simulink model "eVTOL_System"  (R2024b)
settings: Solver=FixedStepAuto  StartTime=0.0  StopTime=inf  RelTol=1e-3
undefined symbols (not defined in the file): airspeed, Battery, BCE12, BCE_Set_init, BMS_Controller_State, C, Cell10_P, Cell11_P, Cell12_P, Cell13_P, Cell14_P, Cell15_P, Cell16_P, Cell17_P, Cell18_P, Cell19_P, Cell1_N, Cell1_P, Cell20_P, Cell21_P, Cell22_P, Cell23_P, Cell24_P, Cell2_P, Cell3_P, Cell4_P, Cell5_P, Cell6_P, Cell7_P, Cell8_P, Cell9_P, Charging_State, CityMission, control, controlParams, ControlSampleTime, CriticalTiltAngle, currentFactor, CV_Gain, ddx, ddy, ddz, Device_01, Device_02, DiscIntNeverNeededParam, dx, dy, dz, Earth, env, F, F28379D_ADC_MaxCount, F28379D_ADC_Vmax, FixedWingMission, flightState, Foc_Ki_IxTcpu, Foc_Ki_S, Foc_Kp_I, Foc_Kp_S, fractalcoef ... (+68)
libraries: fl_lib x1115, nesl_utility x617, slrealtimeethercatlib x217, simulink x130, canmsglib x101, speedgoatlib_IO611_obsolete x91, slpidlib x49, mcbcontrolslib x44, slrealtimeutilitieslib x35, speedgoatlib_hdlCoder_IO3xx x31, dspstat3 x24, mcbpositiondecoderlib x12
(part 29 of 31)

== system eVTOL_System/Motor Drive/Controller/Controller_MIL/F28379D Firmware/Controller Algorithm/FOC/Current Control/Control_System/Closed Loop Control/Subsystem ==
  Iab_meas_PU : Inport
  Pos_PU : Inport  Port=2
  Idq_ref_PU : Inport  Port=3
  EnablePWM : Inport  Port=4
  Kp_i : Inport  Port=5
  Ki_ixTcpu : Inport  Port=6
  Clarke Transform : mcbcontrolslib/Clarke Transform  VariantControl=Variant2  PhaseInput=Two inputs  EnPowerInv=off
  Current_Controllers : Subsystem
  Demux : Demux  Outputs=2
  Inverse Park Transform : mcbcontrolslib/Inverse Park Transform  PhaseInput=Two inputs  AxisAlignment=D-axis  ThetaInput=Sine and Cosine electrical position  AngleInput=Per-unit  N_points=1024
  Mux : Mux
  Mux1 : Mux  Inputs=3
  Park Transform : mcbcontrolslib/Park Transform  PhaseInput=Two inputs  AxisAlignment=D-axis  ThetaInput=Sine and Cosine electrical position  AngleInput=Per-unit  N_points=1024
  Sine-Cosine Lookup : mcbcontrolslib/SinCos Embedded Optimized  LabelModeActiveChoice=MCB_Sin  OptforProc=off  ApproximationMethod=None  UserApproxMethod=Lookup  ApproxStatus=None  InterpMethod=Linear point-slope  NumberOfDataPoints=16  NumberOfIterations=11  RemoveProtectionAgainstOutOfRangeInput=off  TableDataTypeStr=Inherit: Inherit via input  AngleInput=Per-unit  ThetaDataType=single  N_points=1024  DatatypeInput=Inherit from input  Datatype=single
  Space Vector Generator : mcbcontrolslib/PWM Reference Generator  inSignal=Valphabeta  modType=SVM: space vector modulation
  Vabc in PU : Outport  VectorParamsAs1DForOutWhenUnconnected=off
  VIdq_debug : Outport  Port=2  VectorParamsAs1DForOutWhenUnconnected=off
  VI_fb : Outport  Port=3
  wires:
  Space Vector Generator/2 -> Mux1/2
  Clarke Transform/2 -> [Ibeta], Park Transform/2
  Idq_ref_PU/1 -> Current_Controllers/3(Idq_ref_PU)
  Park Transform/1 -> Current_Controllers/1(Id)
  Current_Controllers/1(Vd_ref) -> Inverse Park Transform/1
  Clarke Transform/1 -> [Ialpha], Park Transform/1
  Space Vector Generator/1 -> Mux1/1
  Iab_meas_PU/1 -> Demux/1
  Inverse Park Transform/1 -> [Valpha], Space Vector Generator/1
  Sine-Cosine Lookup/2 -> Park Transform/4, [cosTheta]
  Demux/2 -> Clarke Transform/2
  [sinTheta] -> Inverse Park Transform/3
  Park Transform/2 -> Current_Controllers/2(Iq)
  Current_Controllers/3(VIdq) -> VIdq_debug/1
  Mux1/1 -> Vabc in PU/1
  Sine-Cosine Lookup/1 -> Park Transform/3, [sinTheta]
  Demux/1 -> Clarke Transform/1
  Current_Controllers/2(Vq_ref) -> Inverse Park Transform/2
  [cosTheta] -> Inverse Park Transform/4
  Space Vector Generator/3 -> Mux1/3
  EnablePWM/1 -> Current_Controllers/4(EnablePWM)
  [Valpha] -> Mux/1
  Mux/1 -> VI_fb/1
  Pos_PU/1 -> Sine-Cosine Lookup/1
  Inverse Park Transform/2 -> [Vbeta], Space Vector Generator/2
  [Ialpha] -> Mux/3
  [Ibeta] -> Mux/4
  [Vbeta] -> Mux/2
  Ki_ixTcpu/1 -> Current_Controllers/6(Ki_ixTcpu)
  Kp_i/1 -> Current_Controllers/5(Kp_i)

== system eVTOL_System/Motor Drive/Controller/Controller_MIL/F28379D Firmware/Controller Algorithm/FOC/Current Control/Control_System/Open Loop Start-Up/Ramp Generator ==
  Ramp_Time : Inport
  Enable : Inport  Port=2
  Divide : Product  Inputs=*/  RndMeth=Simplest  OutDataTypeStr=Inherit: Same as first input
  NOT : Logic  Operator=NOT  IconShape=distinctive  AllPortsSameDT=off  OutDataTypeStr=boolean
  One : Constant  OutDataTypeStr=single  SampleTime=-1
  Ramp Generator : DiscreteIntegrator  IntegratorMethod=Accumulation: Forward Euler  gainval=1  ExternalReset=sampled level  SampleTime=-1  OutDataTypeStr=single  RndMeth=Simplest  LimitOutput=on  UpperSaturationLimit=1  LowerSaturationLimit=0  ICPrevOutput=DiscIntNeverNeededParam  ICPrevScaledInput=DiscIntNeverNeededParam
  Sample_Time : Gain  Gain=Ts_CPU  RndMeth=Simplest  OutDataTypeStr=Inherit: Same as input
  Ramp : Outport
  wires:
  Divide/1 -> Sample_Time/1
  Ramp Generator/1 -> Ramp/1  "Eps"
  Sample_Time/1 -> Ramp Generator/1
  One/1 -> Divide/1
  Ramp_Time/1 -> Divide/2
  Enable/1 -> NOT/1
  NOT/1 -> Ramp Generator/2

== system eVTOL_System/Motor Drive/Controller1/Controller_MIL/F28379D Firmware/Controller Algorithm/FOC/Current Control/Control_System/Closed Loop Control/Subsystem ==
  Iab_meas_PU : Inport
  Pos_PU : Inport  Port=2
  Idq_ref_PU : Inport  Port=3
  EnablePWM : Inport  Port=4
  Kp_i : Inport  Port=5
  Ki_ixTcpu : Inport  Port=6
  Clarke Transform : mcbcontrolslib/Clarke Transform  VariantControl=Variant2  PhaseInput=Two inputs  EnPowerInv=off
  Current_Controllers : Subsystem
  Demux : Demux  Outputs=2
  Inverse Park Transform : mcbcontrolslib/Inverse Park Transform  PhaseInput=Two inputs  AxisAlignment=D-axis  ThetaInput=Sine and Cosine electrical position  AngleInput=Per-unit  N_points=1024
  Mux : Mux
  Mux1 : Mux  Inputs=3
  Park Transform : mcbcontrolslib/Park Transform  PhaseInput=Two inputs  AxisAlignment=D-axis  ThetaInput=Sine and Cosine electrical position  AngleInput=Per-unit  N_points=1024
  Sine-Cosine Lookup : mcbcontrolslib/SinCos Embedded Optimized  LabelModeActiveChoice=MCB_Sin  OptforProc=off  ApproximationMethod=None  UserApproxMethod=Lookup  ApproxStatus=None  InterpMethod=Linear point-slope  NumberOfDataPoints=16  NumberOfIterations=11  RemoveProtectionAgainstOutOfRangeInput=off  TableDataTypeStr=Inherit: Inherit via input  AngleInput=Per-unit  ThetaDataType=single  N_points=1024  DatatypeInput=Inherit from input  Datatype=single
  Space Vector Generator : mcbcontrolslib/PWM Reference Generator  inSignal=Valphabeta  modType=SVM: space vector modulation
  Vabc in PU : Outport  VectorParamsAs1DForOutWhenUnconnected=off
  VIdq_debug : Outport  Port=2  VectorParamsAs1DForOutWhenUnconnected=off
  VI_fb : Outport  Port=3
  wires:
  Space Vector Generator/2 -> Mux1/2
  Clarke Transform/2 -> [Ibeta], Park Transform/2
  Idq_ref_PU/1 -> Current_Controllers/3(Idq_ref_PU)
  Park Transform/1 -> Current_Controllers/1(Id)
  Current_Controllers/1(Vd_ref) -> Inverse Park Transform/1
  Clarke Transform/1 -> [Ialpha], Park Transform/1
  Space Vector Generator/1 -> Mux1/1
  Iab_meas_PU/1 -> Demux/1
  Inverse Park Transform/1 -> [Valpha], Space Vector Generator/1
  Sine-Cosine Lookup/2 -> Park Transform/4, [cosTheta]
  Demux/2 -> Clarke Transform/2
  [sinTheta] -> Inverse Park Transform/3
  Park Transform/2 -> Current_Controllers/2(Iq)
  Current_Controllers/3(VIdq) -> VIdq_debug/1
  Mux1/1 -> Vabc in PU/1
  Sine-Cosine Lookup/1 -> Park Transform/3, [sinTheta]
  Demux/1 -> Clarke Transform/1
  Current_Controllers/2(Vq_ref) -> Inverse Park Transform/2
  [cosTheta] -> Inverse Park Transform/4
  Space Vector Generator/3 -> Mux1/3
  EnablePWM/1 -> Current_Controllers/4(EnablePWM)
  [Valpha] -> Mux/1
  Mux/1 -> VI_fb/1
  Pos_PU/1 -> Sine-Cosine Lookup/1
  Inverse Park Transform/2 -> [Vbeta], Space Vector Generator/2
  [Ialpha] -> Mux/3
  [Ibeta] -> Mux/4
  [Vbeta] -> Mux/2
  Ki_ixTcpu/1 -> Current_Controllers/6(Ki_ixTcpu)
  Kp_i/1 -> Current_Controllers/5(Kp_i)

== system eVTOL_System/Motor Drive/Controller1/Controller_MIL/F28379D Firmware/Controller Algorithm/FOC/Current Control/Control_System/Open Loop Start-Up/Ramp Generator ==
  Ramp_Time : Inport
  Enable : Inport  Port=2
  Divide : Product  Inputs=*/  RndMeth=Simplest  OutDataTypeStr=Inherit: Same as first input
  NOT : Logic  Operator=NOT  IconShape=distinctive  AllPortsSameDT=off  OutDataTypeStr=boolean
  One : Constant  OutDataTypeStr=single  SampleTime=-1
  Ramp Generator : DiscreteIntegrator  IntegratorMethod=Accumulation: Forward Euler  gainval=1  ExternalReset=sampled level  SampleTime=-1  OutDataTypeStr=single  RndMeth=Simplest  LimitOutput=on  UpperSaturationLimit=1  LowerSaturationLimit=0  ICPrevOutput=DiscIntNeverNeededParam  ICPrevScaledInput=DiscIntNeverNeededParam
  Sample_Time : Gain  Gain=Ts_CPU  RndMeth=Simplest  OutDataTypeStr=Inherit: Same as input
  Ramp : Outport
  wires:
  Divide/1 -> Sample_Time/1
  Ramp Generator/1 -> Ramp/1  "Eps"
  Sample_Time/1 -> Ramp Generator/1
  One/1 -> Divide/1
  Ramp_Time/1 -> Divide/2
  Enable/1 -> NOT/1
  NOT/1 -> Ramp Generator/2

== system eVTOL_System/Motor Drive/Controller2/Controller_MIL/F28379D Firmware/Controller Algorithm/FOC/Current Control/Control_System/Closed Loop Control/Subsystem ==
  Iab_meas_PU : Inport
  Pos_PU : Inport  Port=2
  Idq_ref_PU : Inport  Port=3
  EnablePWM : Inport  Port=4
  Kp_i : Inport  Port=5
  Ki_ixTcpu : Inport  Port=6
  Clarke Transform : mcbcontrolslib/Clarke Transform  VariantControl=Variant2  PhaseInput=Two inputs  EnPowerInv=off
  Current_Controllers : Subsystem
  Demux : Demux  Outputs=2
  Inverse Park Transform : mcbcontrolslib/Inverse Park Transform  PhaseInput=Two inputs  AxisAlignment=D-axis  ThetaInput=Sine and Cosine electrical position  AngleInput=Per-unit  N_points=1024
  Mux : Mux
  Mux1 : Mux  Inputs=3
  Park Transform : mcbcontrolslib/Park Transform  PhaseInput=Two inputs  AxisAlignment=D-axis  ThetaInput=Sine and Cosine electrical position  AngleInput=Per-unit  N_points=1024
  Sine-Cosine Lookup : mcbcontrolslib/SinCos Embedded Optimized  LabelModeActiveChoice=MCB_Sin  OptforProc=off  ApproximationMethod=None  UserApproxMethod=Lookup  ApproxStatus=None  InterpMethod=Linear point-slope  NumberOfDataPoints=16  NumberOfIterations=11  RemoveProtectionAgainstOutOfRangeInput=off  TableDataTypeStr=Inherit: Inherit via input  AngleInput=Per-unit  ThetaDataType=single  N_points=1024  DatatypeInput=Inherit from input  Datatype=single
  Space Vector Generator : mcbcontrolslib/PWM Reference Generator  inSignal=Valphabeta  modType=SVM: space vector modulation
  Vabc in PU : Outport  VectorParamsAs1DForOutWhenUnconnected=off
  VIdq_debug : Outport  Port=2  VectorParamsAs1DForOutWhenUnconnected=off
  VI_fb : Outport  Port=3
  wires:
  Space Vector Generator/2 -> Mux1/2
  Clarke Transform/2 -> [Ibeta], Park Transform/2
  Idq_ref_PU/1 -> Current_Controllers/3(Idq_ref_PU)
  Park Transform/1 -> Current_Controllers/1(Id)
  Current_Controllers/1(Vd_ref) -> Inverse Park Transform/1
  Clarke Transform/1 -> [Ialpha], Park Transform/1
  Space Vector Generator/1 -> Mux1/1
  Iab_meas_PU/1 -> Demux/1
  Inverse Park Transform/1 -> [Valpha], Space Vector Generator/1
  Sine-Cosine Lookup/2 -> Park Transform/4, [cosTheta]
  Demux/2 -> Clarke Transform/2
  [sinTheta] -> Inverse Park Transform/3
  Park Transform/2 -> Current_Controllers/2(Iq)
  Current_Controllers/3(VIdq) -> VIdq_debug/1
  Mux1/1 -> Vabc in PU/1
  Sine-Cosine Lookup/1 -> Park Transform/3, [sinTheta]
  Demux/1 -> Clarke Transform/1
  Current_Controllers/2(Vq_ref) -> Inverse Park Transform/2
  [cosTheta] -> Inverse Park Transform/4
  Space Vector Generator/3 -> Mux1/3
  EnablePWM/1 -> Current_Controllers/4(EnablePWM)
  [Valpha] -> Mux/1
  Mux/1 -> VI_fb/1
  Pos_PU/1 -> Sine-Cosine Lookup/1
  Inverse Park Transform/2 -> [Vbeta], Space Vector Generator/2
  [Ialpha] -> Mux/3
  [Ibeta] -> Mux/4
  [Vbeta] -> Mux/2
  Ki_ixTcpu/1 -> Current_Controllers/6(Ki_ixTcpu)
  Kp_i/1 -> Current_Controllers/5(Kp_i)

== system eVTOL_System/Motor Drive/Controller2/Controller_MIL/F28379D Firmware/Controller Algorithm/FOC/Current Control/Control_System/Open Loop Start-Up/Ramp Generator ==
  Ramp_Time : Inport
  Enable : Inport  Port=2
  Divide : Product  Inputs=*/  RndMeth=Simplest  OutDataTypeStr=Inherit: Same as first input
  NOT : Logic  Operator=NOT  IconShape=distinctive  AllPortsSameDT=off  OutDataTypeStr=boolean
  One : Constant  OutDataTypeStr=single  SampleTime=-1
  Ramp Generator : DiscreteIntegrator  IntegratorMethod=Accumulation: Forward Euler  gainval=1  ExternalReset=sampled level  SampleTime=-1  OutDataTypeStr=single  RndMeth=Simplest  LimitOutput=on  UpperSaturationLimit=1  LowerSaturationLimit=0  ICPrevOutput=DiscIntNeverNeededParam  ICPrevScaledInput=DiscIntNeverNeededParam
  Sample_Time : Gain  Gain=Ts_CPU  RndMeth=Simplest  OutDataTypeStr=Inherit: Same as input
  Ramp : Outport
  wires:
  Divide/1 -> Sample_Time/1
  Ramp Generator/1 -> Ramp/1  "Eps"
  Sample_Time/1 -> Ramp Generator/1
  One/1 -> Divide/1
  Ramp_Time/1 -> Divide/2
  Enable/1 -> NOT/1
  NOT/1 -> Ramp Generator/2

== system eVTOL_System/Motor Drive/Controller3/Controller_MIL/F28379D Firmware/Controller Algorithm/FOC/Current Control/Control_System/Closed Loop Control/Subsystem ==
  Iab_meas_PU : Inport
  Pos_PU : Inport  Port=2
  Idq_ref_PU : Inport  Port=3
  EnablePWM : Inport  Port=4
  Kp_i : Inport  Port=5
  Ki_ixTcpu : Inport  Port=6
  Clarke Transform : mcbcontrolslib/Clarke Transform  VariantControl=Variant2  PhaseInput=Two inputs  EnPowerInv=off
  Current_Controllers : Subsystem
  Demux : Demux  Outputs=2
  Inverse Park Transform : mcbcontrolslib/Inverse Park Transform  PhaseInput=Two inputs  AxisAlignment=D-axis  ThetaInput=Sine and Cosine electrical position  AngleInput=Per-unit  N_points=1024
  Mux : Mux
  Mux1 : Mux  Inputs=3
  Park Transform : mcbcontrolslib/Park Transform  PhaseInput=Two inputs  AxisAlignment=D-axis  ThetaInput=Sine and Cosine electrical position  AngleInput=Per-unit  N_points=1024
  Sine-Cosine Lookup : mcbcontrolslib/SinCos Embedded Optimized  LabelModeActiveChoice=MCB_Sin  OptforProc=off  ApproximationMethod=None  UserApproxMethod=Lookup  ApproxStatus=None  InterpMethod=Linear point-slope  NumberOfDataPoints=16  NumberOfIterations=11  RemoveProtectionAgainstOutOfRangeInput=off  TableDataTypeStr=Inherit: Inherit via input  AngleInput=Per-unit  ThetaDataType=single  N_points=1024  DatatypeInput=Inherit from input  Datatype=single
  Space Vector Generator : mcbcontrolslib/PWM Reference Generator  inSignal=Valphabeta  modType=SVM: space vector modulation
  Vabc in PU : Outport  VectorParamsAs1DForOutWhenUnconnected=off
  VIdq_debug : Outport  Port=2  VectorParamsAs1DForOutWhenUnconnected=off
  VI_fb : Outport  Port=3
  wires:
  Space Vector Generator/2 -> Mux1/2
  Clarke Transform/2 -> [Ibeta], Park Transform/2
  Idq_ref_PU/1 -> Current_Controllers/3(Idq_ref_PU)
  Park Transform/1 -> Current_Controllers/1(Id)
  Current_Controllers/1(Vd_ref) -> Inverse Park Transform/1
  Clarke Transform/1 -> [Ialpha], Park Transform/1
  Space Vector Generator/1 -> Mux1/1
  Iab_meas_PU/1 -> Demux/1
  Inverse Park Transform/1 -> [Valpha], Space Vector Generator/1
  Sine-Cosine Lookup/2 -> Park Transform/4, [cosTheta]
  Demux/2 -> Clarke Transform/2
  [sinTheta] -> Inverse Park Transform/3
  Park Transform/2 -> Current_Controllers/2(Iq)
  Current_Controllers/3(VIdq) -> VIdq_debug/1
  Mux1/1 -> Vabc in PU/1
  Sine-Cosine Lookup/1 -> Park Transform/3, [sinTheta]
  Demux/1 -> Clarke Transform/1
  Current_Controllers/2(Vq_ref) -> Inverse Park Transform/2
  [cosTheta] -> Inverse Park Transform/4
  Space Vector Generator/3 -> Mux1/3
  EnablePWM/1 -> Current_Controllers/4(EnablePWM)
  [Valpha] -> Mux/1
  Mux/1 -> VI_fb/1
  Pos_PU/1 -> Sine-Cosine Lookup/1
  Inverse Park Transform/2 -> [Vbeta], Space Vector Generator/2
  [Ialpha] -> Mux/3
  [Ibeta] -> Mux/4
  [Vbeta] -> Mux/2
  Ki_ixTcpu/1 -> Current_Controllers/6(Ki_ixTcpu)
  Kp_i/1 -> Current_Controllers/5(Kp_i)

== system eVTOL_System/Motor Drive/Controller3/Controller_MIL/F28379D Firmware/Controller Algorithm/FOC/Current Control/Control_System/Open Loop Start-Up/Ramp Generator ==
  Ramp_Time : Inport
  Enable : Inport  Port=2
  Divide : Product  Inputs=*/  RndMeth=Simplest  OutDataTypeStr=Inherit: Same as first input
  NOT : Logic  Operator=NOT  IconShape=distinctive  AllPortsSameDT=off  OutDataTypeStr=boolean
  One : Constant  OutDataTypeStr=single  SampleTime=-1
  Ramp Generator : DiscreteIntegrator  IntegratorMethod=Accumulation: Forward Euler  gainval=1  ExternalReset=sampled level  SampleTime=-1  OutDataTypeStr=single  RndMeth=Simplest  LimitOutput=on  UpperSaturationLimit=1  LowerSaturationLimit=0  ICPrevOutput=DiscIntNeverNeededParam  ICPrevScaledInput=DiscIntNeverNeededParam
  Sample_Time : Gain  Gain=Ts_CPU  RndMeth=Simplest  OutDataTypeStr=Inherit: Same as input
  Ramp : Outport
  wires:
  Divide/1 -> Sample_Time/1
  Ramp Generator/1 -> Ramp/1  "Eps"
  Sample_Time/1 -> Ramp Generator/1
  One/1 -> Divide/1
  Ramp_Time/1 -> Divide/2
  Enable/1 -> NOT/1
  NOT/1 -> Ramp Generator/2

== system eVTOL_System/Motor Drive/Controller/Controller_MIL/F28379D Firmware/Controller Algorithm/FOC/Current Control/Control_System/Closed Loop Control/Subsystem/Current_Controllers ==
  Id : Inport
  Iq : Inport  Port=2
  Idq_ref_PU : Inport  Port=3
  EnablePWM : Inport  Port=4
  Kp_i : Inport  Port=5
  Ki_ixTcpu : Inport  Port=6
  1/VDC : Gain  Commented=on  Gain=1/((24*sqrt(2/3))*2)
  Bus Creator : BusCreator  Inputs=6
  Constant : Constant  Commented=on  Value=400
  DQ Limiter : mcbcontrolslib/DQ Limiter  satMethodInputType=Specify via dialog  satMethodSelected=D-Q equivalence  satLimitInputType=Specify via dialog  Vmax=0.95
  Demux : Demux  Outputs=2
  Divide : Product  Commented=on  Inputs=*/
  Divide1 : Product  Commented=on  Inputs=*/
  From : From  Commented=on  GotoTag=Voltage  TagVisibility=global
  PI_Controller_Id : Subsystem
  PI_Controller_Iq : Subsystem
  Terminator : Terminator
  Vd_ref : Outport  VectorParamsAs1DForOutWhenUnconnected=off
  Vq_ref : Outport  Port=2  VectorParamsAs1DForOutWhenUnconnected=off
  VIdq : Outport  Port=3  VectorParamsAs1DForOutWhenUnconnected=off
  wires:
  Iq/1 -> Bus Creator/5, PI_Controller_Iq/2(I_fb)  "Iq_fb"
  Id/1 -> PI_Controller_Id/2(I_fb), Bus Creator/2  "Id_fb"
  Demux/1 -> PI_Controller_Id/1(I_ref), Bus Creator/1  "Id_Ref"
  Demux/2 -> Bus Creator/4, PI_Controller_Iq/1(I_ref)  "Iq_Ref"
  Idq_ref_PU/1 -> Demux/1
  DQ Limiter/1 -> Vd_ref/1, Bus Creator/3  "Vd_ref"
  DQ Limiter/2 -> Vq_ref/1, Bus Creator/6  "Vq_ref"
  DQ Limiter/3 -> Terminator/1
  Bus Creator/1 -> VIdq/1
  EnablePWM/1 -> PI_Controller_Iq/3(EnablePWM), PI_Controller_Id/3(EnablePWM)
  Kp_i/1 -> PI_Controller_Iq/4(Kp_i), PI_Controller_Id/4(Kp_i)
  Ki_ixTcpu/1 -> PI_Controller_Iq/5(Ki_ixTcpu), PI_Controller_Id/5(Ki_ixTcpu)
  1/VDC/1 -> Divide/2, Divide1/2
  From/1 -> ?
  Constant/1 -> 1/VDC/1
  PI_Controller_Id/1(V_ref) -> DQ Limiter/1
  PI_Controller_Iq/1(V_ref) -> DQ Limiter/2

== system eVTOL_System/Motor Drive/Controller1/Controller_MIL/F28379D Firmware/Controller Algorithm/FOC/Current Control/Control_System/Closed Loop Control/Subsystem/Current_Controllers ==
  Id : Inport
  Iq : Inport  Port=2
  Idq_ref_PU : Inport  Port=3
  EnablePWM : Inport  Port=4
  Kp_i : Inport  Port=5
  Ki_ixTcpu : Inport  Port=6
  1/VDC : Gain  Commented=on  Gain=1/((24*sqrt(2/3))*2)
  Bus Creator : BusCreator  Inputs=6
  Constant : Constant  Commented=on  Value=400
  DQ Limiter : mcbcontrolslib/DQ Limiter  satMethodInputType=Specify via dialog  satMethodSelected=D-Q equivalence  satLimitInputType=Specify via dialog  Vmax=0.95
  Demux : Demux  Outputs=2
  Divide : Product  Commented=on  Inputs=*/
  Divide1 : Product  Commented=on  Inputs=*/
  From : From  Commented=on  GotoTag=Voltage  TagVisibility=global
  PI_Controller_Id : Subsystem
  PI_Controller_Iq : Subsystem
  Terminator : Terminator
  Vd_ref : Outport  VectorParamsAs1DForOutWhenUnconnected=off
  Vq_ref : Outport  Port=2  VectorParamsAs1DForOutWhenUnconnected=off
  VIdq : Outport  Port=3  VectorParamsAs1DForOutWhenUnconnected=off
  wires:
  Iq/1 -> Bus Creator/5, PI_Controller_Iq/2(I_fb)  "Iq_fb"
  Id/1 -> PI_Controller_Id/2(I_fb), Bus Creator/2  "Id_fb"
  Demux/1 -> PI_Controller_Id/1(I_ref), Bus Creator/1  "Id_Ref"
  Demux/2 -> Bus Creator/4, PI_Controller_Iq/1(I_ref)  "Iq_Ref"
  Idq_ref_PU/1 -> Demux/1
  DQ Limiter/1 -> Vd_ref/1, Bus Creator/3  "Vd_ref"
  DQ Limiter/2 -> Vq_ref/1, Bus Creator/6  "Vq_ref"
  DQ Limiter/3 -> Terminator/1
  Bus Creator/1 -> VIdq/1
  EnablePWM/1 -> PI_Controller_Iq/3(EnablePWM), PI_Controller_Id/3(EnablePWM)
  Kp_i/1 -> PI_Controller_Iq/4(Kp_i), PI_Controller_Id/4(Kp_i)
  Ki_ixTcpu/1 -> PI_Controller_Iq/5(Ki_ixTcpu), PI_Controller_Id/5(Ki_ixTcpu)
  1/VDC/1 -> Divide/2, Divide1/2
  From/1 -> ?
  Constant/1 -> 1/VDC/1
  PI_Controller_Id/1(V_ref) -> DQ Limiter/1
  PI_Controller_Iq/1(V_ref) -> DQ Limiter/2

== system eVTOL_System/Motor Drive/Controller2/Controller_MIL/F28379D Firmware/Controller Algorithm/FOC/Current Control/Control_System/Closed Loop Control/Subsystem/Current_Controllers ==
  Id : Inport
  Iq : Inport  Port=2
  Idq_ref_PU : Inport  Port=3
  EnablePWM : Inport  Port=4
  Kp_i : Inport  Port=5
  Ki_ixTcpu : Inport  Port=6
  1/VDC : Gain  Commented=on  Gain=1/((24*sqrt(2/3))*2)
  Bus Creator : BusCreator  Inputs=6
  Constant : Constant  Commented=on  Value=400
  DQ Limiter : mcbcontrolslib/DQ Limiter  satMethodInputType=Specify via dialog  satMethodSelected=D-Q equivalence  satLimitInputType=Specify via dialog  Vmax=0.95
  Demux : Demux  Outputs=2
  Divide : Product  Commented=on  Inputs=*/
  Divide1 : Product  Commented=on  Inputs=*/
  From : From  Commented=on  GotoTag=Voltage  TagVisibility=global
  PI_Controller_Id : Subsystem
  PI_Controller_Iq : Subsystem
  Terminator : Terminator
  Vd_ref : Outport  VectorParamsAs1DForOutWhenUnconnected=off
  Vq_ref : Outport  Port=2  VectorParamsAs1DForOutWhenUnconnected=off
  VIdq : Outport  Port=3  VectorParamsAs1DForOutWhenUnconnected=off
  wires:
  Iq/1 -> Bus Creator/5, PI_Controller_Iq/2(I_fb)  "Iq_fb"
  Id/1 -> PI_Controller_Id/2(I_fb), Bus Creator/2  "Id_fb"
  Demux/1 -> PI_Controller_Id/1(I_ref), Bus Creator/1  "Id_Ref"
  Demux/2 -> Bus Creator/4, PI_Controller_Iq/1(I_ref)  "Iq_Ref"
  Idq_ref_PU/1 -> Demux/1
  DQ Limiter/1 -> Vd_ref/1, Bus Creator/3  "Vd_ref"
  DQ Limiter/2 -> Vq_ref/1, Bus Creator/6  "Vq_ref"
  DQ Limiter/3 -> Terminator/1
  Bus Creator/1 -> VIdq/1
  EnablePWM/1 -> PI_Controller_Iq/3(EnablePWM), PI_Controller_Id/3(EnablePWM)
  Kp_i/1 -> PI_Controller_Iq/4(Kp_i), PI_Controller_Id/4(Kp_i)
  Ki_ixTcpu/1 -> PI_Controller_Iq/5(Ki_ixTcpu), PI_Controller_Id/5(Ki_ixTcpu)
  1/VDC/1 -> Divide/2, Divide1/2
  From/1 -> ?
  Constant/1 -> 1/VDC/1
  PI_Controller_Id/1(V_ref) -> DQ Limiter/1
  PI_Controller_Iq/1(V_ref) -> DQ Limiter/2

== system eVTOL_System/Motor Drive/Controller3/Controller_MIL/F28379D Firmware/Controller Algorithm/FOC/Current Control/Control_System/Closed Loop Control/Subsystem/Current_Controllers ==
  Id : Inport
  Iq : Inport  Port=2
  Idq_ref_PU : Inport  Port=3
  EnablePWM : Inport  Port=4
  Kp_i : Inport  Port=5
  Ki_ixTcpu : Inport  Port=6
  1/VDC : Gain  Commented=on  Gain=1/((24*sqrt(2/3))*2)
  Bus Creator : BusCreator  Inputs=6
  Constant : Constant  Commented=on  Value=400
  DQ Limiter : mcbcontrolslib/DQ Limiter  satMethodInputType=Specify via dialog  satMethodSelected=D-Q equivalence  satLimitInputType=Specify via dialog  Vmax=0.95
  Demux : Demux  Outputs=2
  Divide : Product  Commented=on  Inputs=*/
  Divide1 : Product  Commented=on  Inputs=*/
  From : From  Commented=on  GotoTag=Voltage  TagVisibility=global
  PI_Controller_Id : Subsystem
  PI_Controller_Iq : Subsystem
  Terminator : Terminator
  Vd_ref : Outport  VectorParamsAs1DForOutWhenUnconnected=off
  Vq_ref : Outport  Port=2  VectorParamsAs1DForOutWhenUnconnected=off
  VIdq : Outport  Port=3  VectorParamsAs1DForOutWhenUnconnected=off
  wires:
  Iq/1 -> Bus Creator/5, PI_Controller_Iq/2(I_fb)  "Iq_fb"
  Id/1 -> PI_Controller_Id/2(I_fb), Bus Creator/2  "Id_fb"
  Demux/1 -> PI_Controller_Id/1(I_ref), Bus Creator/1  "Id_Ref"
  Demux/2 -> Bus Creator/4, PI_Controller_Iq/1(I_ref)  "Iq_Ref"
  Idq_ref_PU/1 -> Demux/1
  DQ Limiter/1 -> Vd_ref/1, Bus Creator/3  "Vd_ref"
  DQ Limiter/2 -> Vq_ref/1, Bus Creator/6  "Vq_ref"
  DQ Limiter/3 -> Terminator/1
  Bus Creator/1 -> VIdq/1
  EnablePWM/1 -> PI_Controller_Iq/3(EnablePWM), PI_Controller_Id/3(EnablePWM)
  Kp_i/1 -> PI_Controller_Iq/4(Kp_i), PI_Controller_Id/4(Kp_i)
  Ki_ixTcpu/1 -> PI_Controller_Iq/5(Ki_ixTcpu), PI_Controller_Id/5(Ki_ixTcpu)
  1/VDC/1 -> Divide/2, Divide1/2
  From/1 -> ?
  Constant/1 -> 1/VDC/1
  PI_Controller_Iq/1(V_ref) -> DQ Limiter/2
  PI_Controller_Id/1(V_ref) -> DQ Limiter/1

== system eVTOL_System/Motor Drive/Controller/Controller_MIL/F28379D Firmware/Controller Algorithm/FOC/Current Control/Control_System/Closed Loop Control/Subsystem/Current_Controllers/PI_Controller_Id ==
  I_ref : Inport
  I_fb : Inport  Port=2
  EnablePWM : Inport  Port=3
  Kp_i : Inport  Port=4
  Ki_ixTcpu : Inport  Port=5
  Discrete PI Controller with anti-windup & reset : slpidlib/PID Controller  Controller=PI  Form=Parallel  TimeDomain=Discrete-time  UseExternalTs=off  SampleTime=-1  IntegratorMethod=Forward Euler  FilterMethod=Forward Euler  ControllerParametersSource=external  P=1  I=1  UseKiTs=on  D=0  UseExternalDerivativeSource=off  N=100  UseFilter=on  TunerSelectOption=Transfer Function Based (PID Tuner App)  InitialConditionSource=external  InitialConditionForIntegrator=0  InitialConditionForFilter=0  DifferentiatorICPrevScaledInput=0  ExternalReset=level  TrackingMode=off  Kt=1  LimitOutput=on  SatLimitsSource=internal  UpperSaturationLimit=1  LowerSaturationLimit=-1  LinearizeAsGain=on  AntiWindupMode=clamping  Kb=1  LimitIntegrator=off  UpperIntegratorSaturationLimit=inf  LowerIntegratorSaturationLimit=-inf  RndMeth=Simplest  POutMin=[]  POutMax=[]  IOutMin=[]  IOutMax=[]  DOutMin=[]  DOutMax=[]  NOutMin=[]  NOutMax=[]  SumOutMin=[]  SumOutMax=[]  SaturationOutDataTypeStr=Inherit: Inherit via back propagation  SaturationOutMin=[]  SaturationOutMax=[]  PParamMin=[]  PParamMax=[]  IParamMin=[]  IParamMax=[]  DParamMin=[]  DParamMax=[]  NParamMin=[]  NParamMax=[]  KbParamMin=[]  KbParamMax=[]  KtParamMin=[]  KtParamMax=[]  KbOutMin=[]  KbOutMax=[]  KtOutMin=[]  KtOutMax=[]  IntegratorOutMin=[]  IntegratorOutMax=[]  FilterOutMin=[]  FilterOutMax=[]  SumI1OutMin=[]  SumI1OutMax=[]  SumI2OutMin=[]  SumI2OutMax=[]  SumI3OutMin=[]  SumI3OutMax=[]  SumI4OutMin=[]  SumI4OutMax=[]  SumDOutMin=[]  SumDOutMax=[]  DifferentiatorOutMin=[]  DifferentiatorOutMax=[]  FilterDiffOutCoefMin=[]  FilterDiffOutCoefMax=[]  ReciprocalOutMin=[]  ReciprocalOutMax=[]  SumDenOutMin=[]  SumDenOutMax=[]  SumNumOutMin=[]  SumNumOutMax=[]  DivideOutMin=[]  DivideOutMax=[]  UdiffTsProdOutMin=[]  UdiffTsProdOutMax=[]  NTsProdOutMin=[]  NTsProdOutMax=[]  UintegralTsProdOutMin=[]  UintegralTsProdOutMax=[]  UngainTsProdOutMin=[]  UngainTsProdOutMax=[]  ClampingZeroOutDataTypeStr=Inherit: Inherit via back propagation  ClampingZeroOutMin=[]  ClampingZeroOutMax=[]  FilterDenConstantOutDataTypeStr=Inherit: Inherit via back propagation  FilterDenConstantOutMin=[]  FilterDenConstantOutMax=[]  PCopyOutDataTypeStr=Inherit: Inherit via back propagation  PCopyOutMin=[]  PCopyOutMax=[]  NCopyOutDataTypeStr=Inherit: Inherit via back propagation  NCopyOutMin=[]  NCopyOutMax=[]  IntegratorContinuousStateAttributes=''  IntegratorStateMustResolveToSignalObject=off  IntegratorRTWStateStorageClass=Auto  FilterContinuousStateAttributes=''  FilterStateMustResolveToSignalObject=off  FilterRTWStateStorageClass=Auto  ParallelPVariant=ExternalParameters  IdealPVariant=Disabled  IVariant=ExternalParameters  DVariant=Disabled  IntegratorVariant=Discrete  SatVariant=Enabled  AWVariant=DiscClampingParallel  PCopyVariant=Disabled  TRVariant=Disabled  FdbkBlocksVariant=Forward  IdealPFdbkVariant=Disabled  SatFdbkVariant=Disabled  DerivativeFilterVariant=Disabled  NVariant=Disabled  NCopyVariant=Disabled_SignalSpec  FilterICVariant=Disabled  IntegratorICVariant=ExternalICs  ExternalResetVariant=ExternalReset  TRSumVariant=Passthrough  SumFdbkVariant=Disabled  SumVariant=Sum_PI  TsampFilterVariant=InternalTs  TsampNgainVariant=Passthrough  TsampIntegralVariant=Disabled_SignalSpec  ExternalSaturationOutDataTypeStr=Inherit: Same as second input  DerivativeSourceVariant=Disabled  PreIntVariant=InternalPreInt
  Ki1 : Constant  Value=0  OutDataTypeStr=single  SampleTime=-1
  Logical Operator : Logic  Operator=NOT  IconShape=distinctive  AllPortsSameDT=off  OutDataTypeStr=boolean
  Sum : Sum  Inputs=|+-  OutDataTypeStr=Inherit: Same as first input
  V_ref : Outport  VectorParamsAs1DForOutWhenUnconnected=off
  wires:
  I_ref/1 -> Sum/1
  I_fb/1 -> Sum/2
  Discrete PI Controller with anti-windup & reset/1 -> V_ref/1
  Sum/1 -> Discrete PI Controller with anti-windup & reset/1
  Logical Operator/1 -> Discrete PI Controller with anti-windup & reset/4
  Ki1/1 -> Discrete PI Controller with anti-windup & reset/5
  EnablePWM/1 -> Logical Operator/1
  Kp_i/1 -> Discrete PI Controller with anti-windup & reset/2
  Ki_ixTcpu/1 -> Discrete PI Controller with anti-windup & reset/3

== system eVTOL_System/Motor Drive/Controller/Controller_MIL/F28379D Firmware/Controller Algorithm/FOC/Current Control/Control_System/Closed Loop Control/Subsystem/Current_Controllers/PI_Controller_Iq ==
  I_ref : Inport
  I_fb : Inport  Port=2
  EnablePWM : Inport  Port=3
  Kp_i : Inport  Port=4
  Ki_ixTcpu : Inport  Port=5
  Discrete PI Controller with anti-windup & reset : slpidlib/PID Controller  Controller=PI  Form=Parallel  TimeDomain=Discrete-time  UseExternalTs=off  SampleTime=-1  IntegratorMethod=Forward Euler  FilterMethod=Forward Euler  ControllerParametersSource=external  P=1  I=1  UseKiTs=on  D=0  UseExternalDerivativeSource=off  N=100  UseFilter=on  TunerSelectOption=Transfer Function Based (PID Tuner App)  InitialConditionSource=external  InitialConditionForIntegrator=0  InitialConditionForFilter=0  DifferentiatorICPrevScaledInput=0  ExternalReset=level  TrackingMode=off  Kt=1  LimitOutput=on  SatLimitsSource=internal  UpperSaturationLimit=1  LowerSaturationLimit=-1  LinearizeAsGain=on  AntiWindupMode=clamping  Kb=1  LimitIntegrator=off  UpperIntegratorSaturationLimit=inf  LowerIntegratorSaturationLimit=-inf  RndMeth=Simplest  POutMin=[]  POutMax=[]  IOutMin=[]  IOutMax=[]  DOutMin=[]  DOutMax=[]  NOutMin=[]  NOutMax=[]  SumOutMin=[]  SumOutMax=[]  SaturationOutDataTypeStr=Inherit: Inherit via back propagation  SaturationOutMin=[]  SaturationOutMax=[]  PParamMin=[]  PParamMax=[]  IParamMin=[]  IParamMax=[]  DParamMin=[]  DParamMax=[]  NParamMin=[]  NParamMax=[]  KbParamMin=[]  KbParamMax=[]  KtParamMin=[]  KtParamMax=[]  KbOutMin=[]  KbOutMax=[]  KtOutMin=[]  KtOutMax=[]  IntegratorOutMin=[]  IntegratorOutMax=[]  FilterOutMin=[]  FilterOutMax=[]  SumI1OutMin=[]  SumI1OutMax=[]  SumI2OutMin=[]  SumI2OutMax=[]  SumI3OutMin=[]  SumI3OutMax=[]  SumI4OutMin=[]  SumI4OutMax=[]  SumDOutMin=[]  SumDOutMax=[]  DifferentiatorOutMin=[]  DifferentiatorOutMax=[]  FilterDiffOutCoefMin=[]  FilterDiffOutCoefMax=[]  ReciprocalOutMin=[]  ReciprocalOutMax=[]  SumDenOutMin=[]  SumDenOutMax=[]  SumNumOutMin=[]  SumNumOutMax=[]  DivideOutMin=[]  DivideOutMax=[]  UdiffTsProdOutMin=[]  UdiffTsProdOutMax=[]  NTsProdOutMin=[]  NTsProdOutMax=[]  UintegralTsProdOutMin=[]  UintegralTsProdOutMax=[]  UngainTsProdOutMin=[]  UngainTsProdOutMax=[]  ClampingZeroOutDataTypeStr=Inherit: Inherit via back propagation  ClampingZeroOutMin=[]  ClampingZeroOutMax=[]  FilterDenConstantOutDataTypeStr=Inherit: Inherit via back propagation  FilterDenConstantOutMin=[]  FilterDenConstantOutMax=[]  PCopyOutDataTypeStr=Inherit: Inherit via back propagation  PCopyOutMin=[]  PCopyOutMax=[]  NCopyOutDataTypeStr=Inherit: Inherit via back propagation  NCopyOutMin=[]  NCopyOutMax=[]  IntegratorContinuousStateAttributes=''  IntegratorStateMustResolveToSignalObject=off  IntegratorRTWStateStorageClass=Auto  FilterContinuousStateAttributes=''  FilterStateMustResolveToSignalObject=off  FilterRTWStateStorageClass=Auto  ParallelPVariant=ExternalParameters  IdealPVariant=Disabled  IVariant=ExternalParameters  DVariant=Disabled  IntegratorVariant=Discrete  SatVariant=Enabled  AWVariant=DiscClampingParallel  PCopyVariant=Disabled  TRVariant=Disabled  FdbkBlocksVariant=Forward  IdealPFdbkVariant=Disabled  SatFdbkVariant=Disabled  DerivativeFilterVariant=Disabled  NVariant=Disabled  NCopyVariant=Disabled_SignalSpec  FilterICVariant=Disabled  IntegratorICVariant=ExternalICs  ExternalResetVariant=ExternalReset  TRSumVariant=Passthrough  SumFdbkVariant=Disabled  SumVariant=Sum_PI  TsampFilterVariant=InternalTs  TsampNgainVariant=Passthrough  TsampIntegralVariant=Disabled_SignalSpec  ExternalSaturationOutDataTypeStr=Inherit: Same as second input  DerivativeSourceVariant=Disabled  PreIntVariant=InternalPreInt
  Kp1 : Constant  Value=0  OutDataTypeStr=single  SampleTime=-1
  Logical Operator : Logic  Operator=NOT  IconShape=distinctive  AllPortsSameDT=off  OutDataTypeStr=boolean
  Sum : Sum  Inputs=|+-  OutDataTypeStr=Inherit: Same as first input
  V_ref : Outport  VectorParamsAs1DForOutWhenUnconnected=off
  wires:
  Discrete PI Controller with anti-windup & reset/1 -> V_ref/1
  I_fb/1 -> Sum/2
  I_ref/1 -> Sum/1
  Sum/1 -> Discrete PI Controller with anti-windup & reset/1
  Logical Operator/1 -> Discrete PI Controller with anti-windup & reset/4
  Kp1/1 -> Discrete PI Controller with anti-windup & reset/5
  EnablePWM/1 -> Logical Operator/1
  Kp_i/1 -> Discrete PI Controller with anti-windup & reset/2
  Ki_ixTcpu/1 -> Discrete PI Controller with anti-windup & reset/3

== system eVTOL_System/Motor Drive/Controller1/Controller_MIL/F28379D Firmware/Controller Algorithm/FOC/Current Control/Control_System/Closed Loop Control/Subsystem/Current_Controllers/PI_Controller_Id ==
  I_ref : Inport
  I_fb : Inport  Port=2
  EnablePWM : Inport  Port=3
  Kp_i : Inport  Port=4
  Ki_ixTcpu : Inport  Port=5
  Discrete PI Controller with anti-windup & reset : slpidlib/PID Controller  Controller=PI  Form=Parallel  TimeDomain=Discrete-time  UseExternalTs=off  SampleTime=-1  IntegratorMethod=Forward Euler  FilterMethod=Forward Euler  ControllerParametersSource=external  P=1  I=1  UseKiTs=on  D=0  UseExternalDerivativeSource=off  N=100  UseFilter=on  TunerSelectOption=Transfer Function Based (PID Tuner App)  InitialConditionSource=external  InitialConditionForIntegrator=0  InitialConditionForFilter=0  DifferentiatorICPrevScaledInput=0  ExternalReset=level  TrackingMode=off  Kt=1  LimitOutput=on  SatLimitsSource=internal  UpperSaturationLimit=1  LowerSaturationLimit=-1  LinearizeAsGain=on  AntiWindupMode=clamping  Kb=1  LimitIntegrator=off  UpperIntegratorSaturationLimit=inf  LowerIntegratorSaturationLimit=-inf  RndMeth=Simplest  POutMin=[]  POutMax=[]  IOutMin=[]  IOutMax=[]  DOutMin=[]  DOutMax=[]  NOutMin=[]  NOutMax=[]  SumOutMin=[]  SumOutMax=[]  SaturationOutDataTypeStr=Inherit: Inherit via back propagation  SaturationOutMin=[]  SaturationOutMax=[]  PParamMin=[]  PParamMax=[]  IParamMin=[]  IParamMax=[]  DParamMin=[]  DParamMax=[]  NParamMin=[]  NParamMax=[]  KbParamMin=[]  KbParamMax=[]  KtParamMin=[]  KtParamMax=[]  KbOutMin=[]  KbOutMax=[]  KtOutMin=[]  KtOutMax=[]  IntegratorOutMin=[]  IntegratorOutMax=[]  FilterOutMin=[]  FilterOutMax=[]  SumI1OutMin=[]  SumI1OutMax=[]  SumI2OutMin=[]  SumI2OutMax=[]  SumI3OutMin=[]  SumI3OutMax=[]  SumI4OutMin=[]  SumI4OutMax=[]  SumDOutMin=[]  SumDOutMax=[]  DifferentiatorOutMin=[]  DifferentiatorOutMax=[]  FilterDiffOutCoefMin=[]  FilterDiffOutCoefMax=[]  ReciprocalOutMin=[]  ReciprocalOutMax=[]  SumDenOutMin=[]  SumDenOutMax=[]  SumNumOutMin=[]  SumNumOutMax=[]  DivideOutMin=[]  DivideOutMax=[]  UdiffTsProdOutMin=[]  UdiffTsProdOutMax=[]  NTsProdOutMin=[]  NTsProdOutMax=[]  UintegralTsProdOutMin=[]  UintegralTsProdOutMax=[]  UngainTsProdOutMin=[]  UngainTsProdOutMax=[]  ClampingZeroOutDataTypeStr=Inherit: Inherit via back propagation  ClampingZeroOutMin=[]  ClampingZeroOutMax=[]  FilterDenConstantOutDataTypeStr=Inherit: Inherit via back propagation  FilterDenConstantOutMin=[]  FilterDenConstantOutMax=[]  PCopyOutDataTypeStr=Inherit: Inherit via back propagation  PCopyOutMin=[]  PCopyOutMax=[]  NCopyOutDataTypeStr=Inherit: Inherit via back propagation  NCopyOutMin=[]  NCopyOutMax=[]  IntegratorContinuousStateAttributes=''  IntegratorStateMustResolveToSignalObject=off  IntegratorRTWStateStorageClass=Auto  FilterContinuousStateAttributes=''  FilterStateMustResolveToSignalObject=off  FilterRTWStateStorageClass=Auto  ParallelPVariant=ExternalParameters  IdealPVariant=Disabled  IVariant=ExternalParameters  DVariant=Disabled  IntegratorVariant=Discrete  SatVariant=Enabled  AWVariant=DiscClampingParallel  PCopyVariant=Disabled  TRVariant=Disabled  FdbkBlocksVariant=Forward  IdealPFdbkVariant=Disabled  SatFdbkVariant=Disabled  DerivativeFilterVariant=Disabled  NVariant=Disabled  NCopyVariant=Disabled_SignalSpec  FilterICVariant=Disabled  IntegratorICVariant=ExternalICs  ExternalResetVariant=ExternalReset  TRSumVariant=Passthrough  SumFdbkVariant=Disabled  SumVariant=Sum_PI  TsampFilterVariant=InternalTs  TsampNgainVariant=Passthrough  TsampIntegralVariant=Disabled_SignalSpec  ExternalSaturationOutDataTypeStr=Inherit: Same as second input  DerivativeSourceVariant=Disabled  PreIntVariant=InternalPreInt
  Ki1 : Constant  Value=0  OutDataTypeStr=single  SampleTime=-1
  Logical Operator : Logic  Operator=NOT  IconShape=distinctive  AllPortsSameDT=off  OutDataTypeStr=boolean
  Sum : Sum  Inputs=|+-  OutDataTypeStr=Inherit: Same as first input
  V_ref : Outport  VectorParamsAs1DForOutWhenUnconnected=off
  wires:
  I_ref/1 -> Sum/1
  I_fb/1 -> Sum/2
  Discrete PI Controller with anti-windup & reset/1 -> V_ref/1
  Sum/1 -> Discrete PI Controller with anti-windup & reset/1
  Logical Operator/1 -> Discrete PI Controller with anti-windup & reset/4
  Ki1/1 -> Discrete PI Controller with anti-windup & reset/5
  EnablePWM/1 -> Logical Operator/1
  Kp_i/1 -> Discrete PI Controller with anti-windup & reset/2
  Ki_ixTcpu/1 -> Discrete PI Controller with anti-windup & reset/3

== system eVTOL_System/Motor Drive/Controller1/Controller_MIL/F28379D Firmware/Controller Algorithm/FOC/Current Control/Control_System/Closed Loop Control/Subsystem/Current_Controllers/PI_Controller_Iq ==
  I_ref : Inport
  I_fb : Inport  Port=2
  EnablePWM : Inport  Port=3
  Kp_i : Inport  Port=4
  Ki_ixTcpu : Inport  Port=5
  Discrete PI Controller with anti-windup & reset : slpidlib/PID Controller  Controller=PI  Form=Parallel  TimeDomain=Discrete-time  UseExternalTs=off  SampleTime=-1  IntegratorMethod=Forward Euler  FilterMethod=Forward Euler  ControllerParametersSource=external  P=1  I=1  UseKiTs=on  D=0  UseExternalDerivativeSource=off  N=100  UseFilter=on  TunerSelectOption=Transfer Function Based (PID Tuner App)  InitialConditionSource=external  InitialConditionForIntegrator=0  InitialConditionForFilter=0  DifferentiatorICPrevScaledInput=0  ExternalReset=level  TrackingMode=off  Kt=1  LimitOutput=on  SatLimitsSource=internal  UpperSaturationLimit=1  LowerSaturationLimit=-1  LinearizeAsGain=on  AntiWindupMode=clamping  Kb=1  LimitIntegrator=off  UpperIntegratorSaturationLimit=inf  LowerIntegratorSaturationLimit=-inf  RndMeth=Simplest  POutMin=[]  POutMax=[]  IOutMin=[]  IOutMax=[]  DOutMin=[]  DOutMax=[]  NOutMin=[]  NOutMax=[]  SumOutMin=[]  SumOutMax=[]  SaturationOutDataTypeStr=Inherit: Inherit via back propagation  SaturationOutMin=[]  SaturationOutMax=[]  PParamMin=[]  PParamMax=[]  IParamMin=[]  IParamMax=[]  DParamMin=[]  DParamMax=[]  NParamMin=[]  NParamMax=[]  KbParamMin=[]  KbParamMax=[]  KtParamMin=[]  KtParamMax=[]  KbOutMin=[]  KbOutMax=[]  KtOutMin=[]  KtOutMax=[]  IntegratorOutMin=[]  IntegratorOutMax=[]  FilterOutMin=[]  FilterOutMax=[]  SumI1OutMin=[]  SumI1OutMax=[]  SumI2OutMin=[]  SumI2OutMax=[]  SumI3OutMin=[]  SumI3OutMax=[]  SumI4OutMin=[]  SumI4OutMax=[]  SumDOutMin=[]  SumDOutMax=[]  DifferentiatorOutMin=[]  DifferentiatorOutMax=[]  FilterDiffOutCoefMin=[]  FilterDiffOutCoefMax=[]  ReciprocalOutMin=[]  ReciprocalOutMax=[]  SumDenOutMin=[]  SumDenOutMax=[]  SumNumOutMin=[]  SumNumOutMax=[]  DivideOutMin=[]  DivideOutMax=[]  UdiffTsProdOutMin=[]  UdiffTsProdOutMax=[]  NTsProdOutMin=[]  NTsProdOutMax=[]  UintegralTsProdOutMin=[]  UintegralTsProdOutMax=[]  UngainTsProdOutMin=[]  UngainTsProdOutMax=[]  ClampingZeroOutDataTypeStr=Inherit: Inherit via back propagation  ClampingZeroOutMin=[]  ClampingZeroOutMax=[]  FilterDenConstantOutDataTypeStr=Inherit: Inherit via back propagation  FilterDenConstantOutMin=[]  FilterDenConstantOutMax=[]  PCopyOutDataTypeStr=Inherit: Inherit via back propagation  PCopyOutMin=[]  PCopyOutMax=[]  NCopyOutDataTypeStr=Inherit: Inherit via back propagation  NCopyOutMin=[]  NCopyOutMax=[]  IntegratorContinuousStateAttributes=''  IntegratorStateMustResolveToSignalObject=off  IntegratorRTWStateStorageClass=Auto  FilterContinuousStateAttributes=''  FilterStateMustResolveToSignalObject=off  FilterRTWStateStorageClass=Auto  ParallelPVariant=ExternalParameters  IdealPVariant=Disabled  IVariant=ExternalParameters  DVariant=Disabled  IntegratorVariant=Discrete  SatVariant=Enabled  AWVariant=DiscClampingParallel  PCopyVariant=Disabled  TRVariant=Disabled  FdbkBlocksVariant=Forward  IdealPFdbkVariant=Disabled  SatFdbkVariant=Disabled  DerivativeFilterVariant=Disabled  NVariant=Disabled  NCopyVariant=Disabled_SignalSpec  FilterICVariant=Disabled  IntegratorICVariant=ExternalICs  ExternalResetVariant=ExternalReset  TRSumVariant=Passthrough  SumFdbkVariant=Disabled  SumVariant=Sum_PI  TsampFilterVariant=InternalTs  TsampNgainVariant=Passthrough  TsampIntegralVariant=Disabled_SignalSpec  ExternalSaturationOutDataTypeStr=Inherit: Same as second input  DerivativeSourceVariant=Disabled  PreIntVariant=InternalPreInt
  Kp1 : Constant  Value=0  OutDataTypeStr=single  SampleTime=-1
  Logical Operator : Logic  Operator=NOT  IconShape=distinctive  AllPortsSameDT=off  OutDataTypeStr=boolean
  Sum : Sum  Inputs=|+-  OutDataTypeStr=Inherit: Same as first input
  V_ref : Outport  VectorParamsAs1DForOutWhenUnconnected=off
  wires:
  Discrete PI Controller with anti-windup & reset/1 -> V_ref/1
  I_fb/1 -> Sum/2
  I_ref/1 -> Sum/1
  Sum/1 -> Discrete PI Controller with anti-windup & reset/1
  Logical Operator/1 -> Discrete PI Controller with anti-windup & reset/4
  Kp1/1 -> Discrete PI Controller with anti-windup & reset/5
  EnablePWM/1 -> Logical Operator/1
  Kp_i/1 -> Discrete PI Controller with anti-windup & reset/2
  Ki_ixTcpu/1 -> Discrete PI Controller with anti-windup & reset/3

== system eVTOL_System/Motor Drive/Controller2/Controller_MIL/F28379D Firmware/Controller Algorithm/FOC/Current Control/Control_System/Closed Loop Control/Subsystem/Current_Controllers/PI_Controller_Id ==
  I_ref : Inport
  I_fb : Inport  Port=2
  EnablePWM : Inport  Port=3
  Kp_i : Inport  Port=4
  Ki_ixTcpu : Inport  Port=5
  Discrete PI Controller with anti-windup & reset : slpidlib/PID Controller  Controller=PI  Form=Parallel  TimeDomain=Discrete-time  UseExternalTs=off  SampleTime=-1  IntegratorMethod=Forward Euler  FilterMethod=Forward Euler  ControllerParametersSource=external  P=1  I=1  UseKiTs=on  D=0  UseExternalDerivativeSource=off  N=100  UseFilter=on  TunerSelectOption=Transfer Function Based (PID Tuner App)  InitialConditionSource=external  InitialConditionForIntegrator=0  InitialConditionForFilter=0  DifferentiatorICPrevScaledInput=0  ExternalReset=level  TrackingMode=off  Kt=1  LimitOutput=on  SatLimitsSource=internal  UpperSaturationLimit=1  LowerSaturationLimit=-1  LinearizeAsGain=on  AntiWindupMode=clamping  Kb=1  LimitIntegrator=off  UpperIntegratorSaturationLimit=inf  LowerIntegratorSaturationLimit=-inf  RndMeth=Simplest  POutMin=[]  POutMax=[]  IOutMin=[]  IOutMax=[]  DOutMin=[]  DOutMax=[]  NOutMin=[]  NOutMax=[]  SumOutMin=[]  SumOutMax=[]  SaturationOutDataTypeStr=Inherit: Inherit via back propagation  SaturationOutMin=[]  SaturationOutMax=[]  PParamMin=[]  PParamMax=[]  IParamMin=[]  IParamMax=[]  DParamMin=[]  DParamMax=[]  NParamMin=[]  NParamMax=[]  KbParamMin=[]  KbParamMax=[]  KtParamMin=[]  KtParamMax=[]  KbOutMin=[]  KbOutMax=[]  KtOutMin=[]  KtOutMax=[]  IntegratorOutMin=[]  IntegratorOutMax=[]  FilterOutMin=[]  FilterOutMax=[]  SumI1OutMin=[]  SumI1OutMax=[]  SumI2OutMin=[]  SumI2OutMax=[]  SumI3OutMin=[]  SumI3OutMax=[]  SumI4OutMin=[]  SumI4OutMax=[]  SumDOutMin=[]  SumDOutMax=[]  DifferentiatorOutMin=[]  DifferentiatorOutMax=[]  FilterDiffOutCoefMin=[]  FilterDiffOutCoefMax=[]  ReciprocalOutMin=[]  ReciprocalOutMax=[]  SumDenOutMin=[]  SumDenOutMax=[]  SumNumOutMin=[]  SumNumOutMax=[]  DivideOutMin=[]  DivideOutMax=[]  UdiffTsProdOutMin=[]  UdiffTsProdOutMax=[]  NTsProdOutMin=[]  NTsProdOutMax=[]  UintegralTsProdOutMin=[]  UintegralTsProdOutMax=[]  UngainTsProdOutMin=[]  UngainTsProdOutMax=[]  ClampingZeroOutDataTypeStr=Inherit: Inherit via back propagation  ClampingZeroOutMin=[]  ClampingZeroOutMax=[]  FilterDenConstantOutDataTypeStr=Inherit: Inherit via back propagation  FilterDenConstantOutMin=[]  FilterDenConstantOutMax=[]  PCopyOutDataTypeStr=Inherit: Inherit via back propagation  PCopyOutMin=[]  PCopyOutMax=[]  NCopyOutDataTypeStr=Inherit: Inherit via back propagation  NCopyOutMin=[]  NCopyOutMax=[]  IntegratorContinuousStateAttributes=''  IntegratorStateMustResolveToSignalObject=off  IntegratorRTWStateStorageClass=Auto  FilterContinuousStateAttributes=''  FilterStateMustResolveToSignalObject=off  FilterRTWStateStorageClass=Auto  ParallelPVariant=ExternalParameters  IdealPVariant=Disabled  IVariant=ExternalParameters  DVariant=Disabled  IntegratorVariant=Discrete  SatVariant=Enabled  AWVariant=DiscClampingParallel  PCopyVariant=Disabled  TRVariant=Disabled  FdbkBlocksVariant=Forward  IdealPFdbkVariant=Disabled  SatFdbkVariant=Disabled  DerivativeFilterVariant=Disabled  NVariant=Disabled  NCopyVariant=Disabled_SignalSpec  FilterICVariant=Disabled  IntegratorICVariant=ExternalICs  ExternalResetVariant=ExternalReset  TRSumVariant=Passthrough  SumFdbkVariant=Disabled  SumVariant=Sum_PI  TsampFilterVariant=InternalTs  TsampNgainVariant=Passthrough  TsampIntegralVariant=Disabled_SignalSpec  ExternalSaturationOutDataTypeStr=Inherit: Same as second input  DerivativeSourceVariant=Disabled  PreIntVariant=InternalPreInt
  Ki1 : Constant  Value=0  OutDataTypeStr=single  SampleTime=-1
  Logical Operator : Logic  Operator=NOT  IconShape=distinctive  AllPortsSameDT=off  OutDataTypeStr=boolean
  Sum : Sum  Inputs=|+-  OutDataTypeStr=Inherit: Same as first input
  V_ref : Outport  VectorParamsAs1DForOutWhenUnconnected=off
  wires:
  I_ref/1 -> Sum/1
  I_fb/1 -> Sum/2
  Discrete PI Controller with anti-windup & reset/1 -> V_ref/1
  Sum/1 -> Discrete PI Controller with anti-windup & reset/1
  Logical Operator/1 -> Discrete PI Controller with anti-windup & reset/4
  Ki1/1 -> Discrete PI Controller with anti-windup & reset/5
  EnablePWM/1 -> Logical Operator/1
  Kp_i/1 -> Discrete PI Controller with anti-windup & reset/2
  Ki_ixTcpu/1 -> Discrete PI Controller with anti-windup & reset/3
